simulink model "MAIN"  (R2021b)
settings: Solver=VariableStepAuto  StartTime=0.0  StopTime=10  RelTol=1e-3
undefined symbols (not defined in the file): c_Fuel, CM_FUEL_b, cmFuel_cmL, g, k_Fuel, L_TV, m_dot, m_iFuel, sigbuilder_block, T_min, VRfromNED_cordT, W_LANDER
libraries: matrix_library x3, slpidlib x2, shared6dof x1, simulink x1, aerolibanim x1, vrlib x1
settings Model: Creator=josepfamador  LastModifiedBy=josepfamador
settings DebuggingCC: SignalRangeChecking=warning  AlgebraicLoopMsg=none

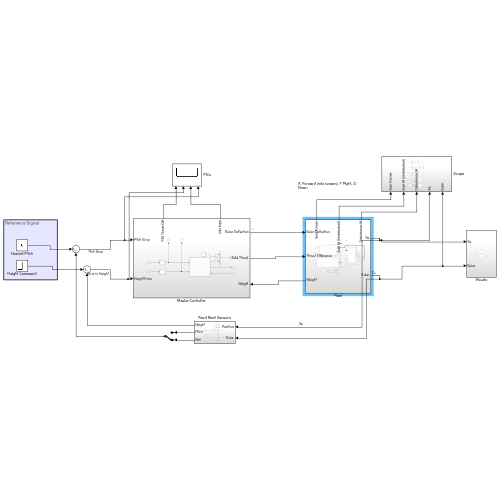
[thumbnail: Simulink's stored preview of the top-level diagram]
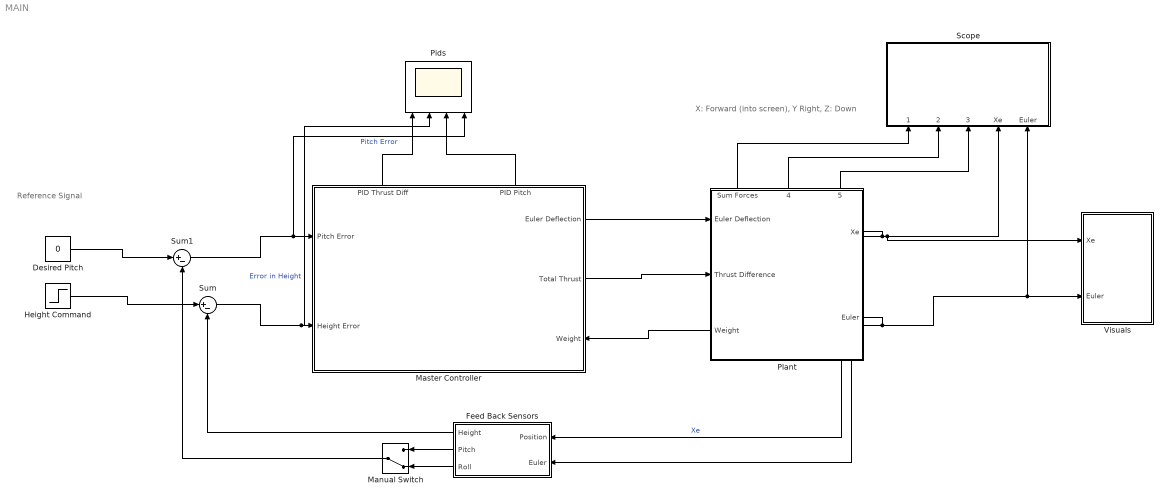
== system MAIN ==
  note: Reference Signal
  note: X: Forward (into screen), Y Right, Z: Down
  Desired Pitch : Constant  Value=0
  Feed Back Sensors : Subsystem
  Height Command : Step  SampleTime=0
  Manual Switch : ManualSwitch  CurrentSetting=0
  Master Controller : Subsystem
      settings: PortSchema="{\"entries\":[{\"content\":{\"sides\":[{\"content\":{\"connectorIds\":[\"In1\",\"In2\"]},\"type\":\"ConnectorPlacement.EquallySpacedRectSide\",\"uuid\":\"6b5f81e2-01db-4c59-bf08-4e3bf18bec3e\"},{\"content\":{\"connectorIds\":[\"Out1\",\"Out2\",\"In3\"],\"side\":\"RIGHT\"},\"type\":\"ConnectorPlacement.EquallySpacedRectSide\",\"uuid\":\"f97d49e1-5da4-4301-bd73-5a99c2855c55\"},{\"content\":{\"connectorIds\":[\"Out3\",\"Out4\"],\"side\":\"TOP\"},\"type\":\"ConnectorPlacement.EquallySpacedRectSide\",\"uuid\":\"d62bb92c-f39d-4cdf-a376-fbc7197c24fb\"}]},\"type\":\"ConnectorPlacement.EquallySpacedConnector\",\"uuid\":\"6638e0f7-5996-4093-84e0-c43993169f29\"}],\"packageUris\":[\"http://schema.mathworks.com/mf0/Connector/R2020b\"],\"version\":\"1.0\"}"
  Pids : Scope  NumInputPorts=4
  Plant : Subsystem
      settings: PortSchema="{\"entries\":[{\"content\":{\"sides\":[{\"content\":{\"connectorIds\":[\"In1\",\"In2\",\"Out6\"]},\"type\":\"ConnectorPlacement.EquallySpacedRectSide\",\"uuid\":\"a758654d-f9c5-4f69-af4d-6756fdff02ab\"},{\"content\":{\"connectorIds\":[\"Out1\",\"Out2\"],\"side\":\"RIGHT\"},\"type\":\"ConnectorPlacement.EquallySpacedRectSide\",\"uuid\":\"3ca0fdf4-fd7f-4f85-961a-cf19d643cdba\"},{\"content\":{\"connectorIds\":[\"Out3\",\"Out4\",\"Out5\"],\"side\":\"TOP\"},\"type\":\"ConnectorPlacement.EquallySpacedRectSide\",\"uuid\":\"8f9619ba-17bf-4a52-b197-69b799ce5fe6\"}]},\"type\":\"ConnectorPlacement.EquallySpacedConnector\",\"uuid\":\"48dcdf5d-501a-46a0-b089-89402a42e7cd\"}],\"packageUris\":[\"http://schema.mathworks.com/mf0/Connector/R2020b\"],\"version\":\"1.0\"}"
  Scope : Subsystem
  Sum : Sum  Inputs=|+-
  Sum1 : Sum  Inputs=|+-
  Visuals : Subsystem
  wires:
  Plant/1(Xe) -> Feed Back Sensors/1(Position), Scope/4(Xe), Visuals/1(Xe)  "Xe"
  Desired Pitch/1 -> Sum1/1
  Height Command/1 -> Sum/1
  Plant/2(Euler) -> Feed Back Sensors/2(Euler), Visuals/2(Euler), Scope/5(Euler)
  Feed Back Sensors/1(Height) -> Sum/2
  Sum1/1 -> Pids/4, Master Controller/1(Pitch Error)  "Pitch Error"
  Sum/1 -> Pids/2, Master Controller/2(Height Error)  "Error in Height"
  Plant/6(Weight) -> Master Controller/3(Weight)
  Master Controller/3(PID Thrust Diff) -> Pids/1
  Master Controller/4(PID Pitch) -> Pids/3
  Master Controller/1(Euler Deflection) -> Plant/1(Euler Deflection)
  Master Controller/2(Total Thrust) -> Plant/2(Thrust Difference)
  Plant/3(Sum Forces) -> Scope/1(Sum Forces)
  Plant/4(Sum M (Undisturbed)) -> Scope/2(Sum M (Undisturbed))
  Plant/5(Disturbance M) -> Scope/3(Disturbance M)
  Feed Back Sensors/3(Roll) -> Manual Switch/2
  Feed Back Sensors/2(Pitch) -> Manual Switch/1
  Manual Switch/1 -> Sum1/2

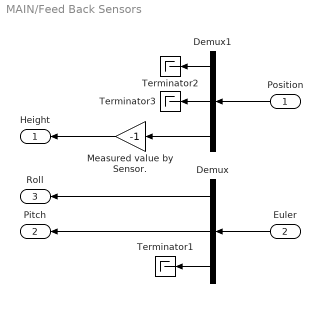
== system MAIN/Feed Back Sensors ==
  Position : Inport
  Euler : Inport  Port=2
  Demux : Demux  Outputs=3
  Demux1 : Demux  Outputs=3
  Measured value by Sensor. : Gain  Gain=-1
  Terminator1 : Terminator
  Terminator2 : Terminator
  Terminator3 : Terminator
  Height : Outport
  Pitch : Outport  Port=2
  Roll : Outport  Port=3
  wires:
  Position/1 -> Demux1/1
  Euler/1 -> Demux/1
  Measured value by Sensor./1 -> Height/1
  Demux/2 -> Pitch/1
  Demux/1 -> Roll/1
  Demux1/2 -> Terminator3/1
  Demux1/1 -> Terminator2/1
  Demux1/3 -> Measured value by Sensor./1
  Demux/3 -> Terminator1/1

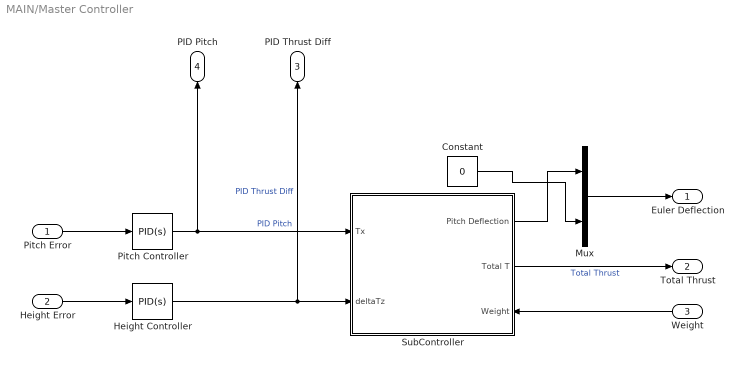
== system MAIN/Master Controller ==
  Pitch Error : Inport
  Height Error : Inport  Port=2
  Weight : Inport  Port=3
  Constant : Constant  Value=0
  Height Controller : slpidlib/PID Controller  Controller=PID  Form=Parallel  TimeDomain=Continuous-time  UseExternalTs=off  SampleTime=-1  IntegratorMethod=Forward Euler  FilterMethod=Forward Euler  ControllerParametersSource=internal  P=32  I=0.2  D=2  UseFilter=on  N=100  TunerSelectOption=Transfer Function Based (PID Tuner App)  InitialConditionSource=internal  InitialConditionForIntegrator=0  InitialConditionForFilter=0  DifferentiatorICPrevScaledInput=0  ExternalReset=none  TrackingMode=off  Kt=1  LimitOutput=on  SatLimitsSource=internal  UpperSaturationLimit=500  LowerSaturationLimit=-inf  LinearizeAsGain=off  AntiWindupMode=none  Kb=1  POutMin=[]  POutMax=[]  IOutMin=[]  IOutMax=[]  DOutMin=[]  DOutMax=[]  NOutMin=[]  NOutMax=[]  SumOutMin=[]  SumOutMax=[]  SaturationOutMin=[]  SaturationOutMax=[]  PParamMin=[]  PParamMax=[]  IParamMin=[]  IParamMax=[]  DParamMin=[]  DParamMax=[]  NParamMin=[]  NParamMax=[]  KbParamMin=[]  KbParamMax=[]  KtParamMin=[]  KtParamMax=[]  KbOutMin=[]  KbOutMax=[]  KtOutMin=[]  KtOutMax=[]  IntegratorOutMin=[]  IntegratorOutMax=[]  FilterOutMin=[]  FilterOutMax=[]  SumI1OutMin=[]  SumI1OutMax=[]  SumI2OutMin=[]  SumI2OutMax=[]  SumI3OutMin=[]  SumI3OutMax=[]  SumI4OutMin=[]  SumI4OutMax=[]  SumDOutMin=[]  SumDOutMax=[]  DifferentiatorOutMin=[]  DifferentiatorOutMax=[]  FilterDiffOutCoefMin=[]  FilterDiffOutCoefMax=[]  ReciprocalOutMin=[]  ReciprocalOutMax=[]  SumDenOutMin=[]  SumDenOutMax=[]  SumNumOutMin=[]  SumNumOutMax=[]  DivideOutMin=[]  DivideOutMax=[]  UdiffTsProdOutMin=[]  UdiffTsProdOutMax=[]  NTsProdOutMin=[]  NTsProdOutMax=[]  UintegralTsProdOutMin=[]  UintegralTsProdOutMax=[]  UngainTsProdOutMin=[]  UngainTsProdOutMax=[]  IntegratorContinuousStateAttributes=''  IntegratorStateMustResolveToSignalObject=off  IntegratorRTWStateStorageClass=Auto  FilterContinuousStateAttributes=''  FilterStateMustResolveToSignalObject=off  FilterRTWStateStorageClass=Auto  ParallelPVariant=InternalParameters  IdealPVariant=Disabled  IVariant=InternalParameters  DVariant=InternalParameters  IntegratorVariant=Continuous  SatVariant=Enabled  AWVariant=Passthrough  PCopyVariant=Disabled  TRVariant=Disabled  FdbkBlocksVariant=Forward  IdealPFdbkVariant=Disabled  SatFdbkVariant=Disabled  DerivativeFilterVariant=ContFilter  NVariant=InternalParameters  NCopyVariant=Disabled  FilterICVariant=InternalICsFilter  IntegratorICVariant=InternalICs  ExternalResetVariant=Disabled  TRSumVariant=Passthrough  SumFdbkVariant=Disabled  SumVariant=Sum_PID  TsampFilterVariant=InternalTs  TsampNgainVariant=Passthrough  TsampIntegralVariant=Passthrough  ExternalSaturationOutDataTypeStr=Inherit: Same as second input
  Mux : Mux  Inputs=2
  Pitch Controller : slpidlib/PID Controller  Controller=PID  Form=Parallel  TimeDomain=Continuous-time  UseExternalTs=off  SampleTime=-1  IntegratorMethod=Forward Euler  FilterMethod=Forward Euler  ControllerParametersSource=internal  P=-0.5002  I=0  D=0  UseFilter=on  N=100  TunerSelectOption=Frequency Response Based  InitialConditionSource=internal  InitialConditionForIntegrator=0  InitialConditionForFilter=0  DifferentiatorICPrevScaledInput=0  ExternalReset=none  TrackingMode=off  Kt=1  LimitOutput=on  SatLimitsSource=internal  UpperSaturationLimit=0.2618  LowerSaturationLimit=-0.2618  LinearizeAsGain=on  AntiWindupMode=none  Kb=1  POutMin=[]  POutMax=[]  IOutMin=[]  IOutMax=[]  DOutMin=[]  DOutMax=[]  NOutMin=[]  NOutMax=[]  SumOutMin=[]  SumOutMax=[]  SaturationOutMin=[]  SaturationOutMax=[]  PParamMin=[]  PParamMax=[]  IParamMin=[]  IParamMax=[]  DParamMin=[]  DParamMax=[]  NParamMin=[]  NParamMax=[]  KbParamMin=[]  KbParamMax=[]  KtParamMin=[]  KtParamMax=[]  KbOutMin=[]  KbOutMax=[]  KtOutMin=[]  KtOutMax=[]  IntegratorOutMin=[]  IntegratorOutMax=[]  FilterOutMin=[]  FilterOutMax=[]  SumI1OutMin=[]  SumI1OutMax=[]  SumI2OutMin=[]  SumI2OutMax=[]  SumI3OutMin=[]  SumI3OutMax=[]  SumI4OutMin=[]  SumI4OutMax=[]  SumDOutMin=[]  SumDOutMax=[]  DifferentiatorOutMin=[]  DifferentiatorOutMax=[]  FilterDiffOutCoefMin=[]  FilterDiffOutCoefMax=[]  ReciprocalOutMin=[]  ReciprocalOutMax=[]  SumDenOutMin=[]  SumDenOutMax=[]  SumNumOutMin=[]  SumNumOutMax=[]  DivideOutMin=[]  DivideOutMax=[]  UdiffTsProdOutMin=[]  UdiffTsProdOutMax=[]  NTsProdOutMin=[]  NTsProdOutMax=[]  UintegralTsProdOutMin=[]  UintegralTsProdOutMax=[]  UngainTsProdOutMin=[]  UngainTsProdOutMax=[]  IntegratorContinuousStateAttributes=''  IntegratorStateMustResolveToSignalObject=off  IntegratorRTWStateStorageClass=Auto  FilterContinuousStateAttributes=''  FilterStateMustResolveToSignalObject=off  FilterRTWStateStorageClass=Auto  ParallelPVariant=InternalParameters  IdealPVariant=Disabled  IVariant=InternalParameters  DVariant=InternalParameters  IntegratorVariant=Continuous  SatVariant=Enabled  AWVariant=Passthrough  PCopyVariant=Disabled  TRVariant=Disabled  FdbkBlocksVariant=Forward  IdealPFdbkVariant=Disabled  SatFdbkVariant=Disabled  DerivativeFilterVariant=ContFilter  NVariant=InternalParameters  NCopyVariant=Disabled  FilterICVariant=InternalICsFilter  IntegratorICVariant=InternalICs  ExternalResetVariant=Disabled  TRSumVariant=Passthrough  SumFdbkVariant=Disabled  SumVariant=Sum_PID  TsampFilterVariant=InternalTs  TsampNgainVariant=Passthrough  TsampIntegralVariant=Passthrough  ExternalSaturationOutDataTypeStr=Inherit: Same as second input
  SubController : Subsystem
      settings: PortSchema="{\"entries\":[{\"content\":{\"sides\":[{\"content\":{\"connectorIds\":[\"In1\",\"In2\"]},\"type\":\"ConnectorPlacement.EquallySpacedRectSide\",\"uuid\":\"09ce5825-295e-43a7-9644-a5328231df2c\"},{\"content\":{\"connectorIds\":[\"Out1\",\"Out2\",\"In3\"],\"side\":\"RIGHT\"},\"type\":\"ConnectorPlacement.EquallySpacedRectSide\",\"uuid\":\"578e798d-aacd-4cff-b78a-042079318f31\"},{\"content\":{\"connectorIds\":[],\"side\":\"TOP\"},\"type\":\"ConnectorPlacement.EquallySpacedRectSide\",\"uuid\":\"66791839-dddf-41e6-aa5f-32841b466e1e\"}]},\"type\":\"ConnectorPlacement.EquallySpacedConnector\",\"uuid\":\"3e01a88c-8ac0-4240-97e5-f19006a6fa45\"}],\"packageUris\":[\"http://schema.mathworks.com/mf0/Connector/R2020b\"],\"version\":\"1.0\"}"
  Euler Deflection : Outport
  Total Thrust : Outport  Port=2
  PID Thrust Diff : Outport  Port=3
  PID Pitch : Outport  Port=4
  wires:
  Mux/1 -> Euler Deflection/1
  Height Error/1 -> Height Controller/1
  Weight/1 -> SubController/3(Weight)
  SubController/2(Total T) -> Total Thrust/1  "Total Thrust"
  Height Controller/1 -> SubController/2(deltaTz), PID Thrust Diff/1  "PID Thrust Diff"
  Pitch Controller/1 -> SubController/1(Tx), PID Pitch/1  "PID Pitch"
  Pitch Error/1 -> Pitch Controller/1
  SubController/1(Pitch Deflection) -> Mux/1
  Constant/1 -> Mux/2

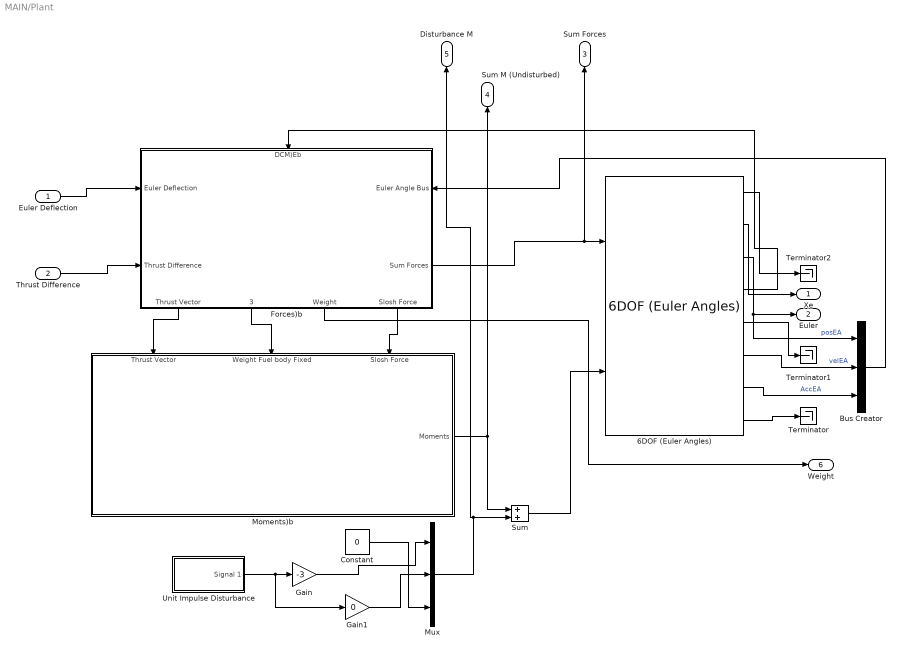
== system MAIN/Plant ==
  Euler Deflection : Inport
  Thrust Difference : Inport  Port=2
  6DOF (Euler Angles) : shared6dof/6DOF (Euler Angles)  units=Metric (MKS)  mtype=Fixed  rep=Euler Angles  xme_0=[0 0 0]  Vm_0=[0 0 0]  eul_0=[0 0 0]  pm_0=[0 0 0]  mass_0=M_lander  mass_e=0.5  mass_f=2.0  inertia=I  inertia_e=eye(3)  inertia_f=2*eye(3)  k_quat=1.0  vre_flag=on  abi_flag=off  aMode=0  xme_statename=''  Vm_statename=''  eul_statename=''  quat_statename=''  pm_statename=''  mass_statename=''
      settings: SourceProductBaseCode=AE,PW,DR,MT,UV,VE
  Bus Creator : BusCreator  Inputs=3
  Constant : Constant  Value=0
  Forces)b : Subsystem
      settings: PortSchema="{\"entries\":[{\"content\":{\"sides\":[{\"content\":{\"connectorIds\":[\"In1\",\"In2\"]},\"type\":\"ConnectorPlacement.EquallySpacedRectSide\",\"uuid\":\"f2cd2bb8-6e5d-4153-a512-e15a3f9d81c4\"},{\"content\":{\"connectorIds\":[\"In4\",\"Out1\"],\"side\":\"RIGHT\"},\"type\":\"ConnectorPlacement.EquallySpacedRectSide\",\"uuid\":\"118a6529-12fa-490e-97a8-013bcc90e0c4\"},{\"content\":{\"connectorIds\":[\"In3\"],\"side\":\"TOP\"},\"type\":\"ConnectorPlacement.EquallySpacedRectSide\",\"uuid\":\"99a35966-8420-41f8-be1a-036ce80ff0d6\"},{\"content\":{\"connectorIds\":[\"Out2\",\"Out3\",\"Out4\",\"Out5\"],\"side\":\"BOTTOM\"},\"type\":\"ConnectorPlacement.EquallySpacedRectSide\",\"uuid\":\"85926175-8560-4c6d-bfea-5508daccda47\"}]},\"type\":\"ConnectorPlacement.EquallySpacedConnector\",\"uuid\":\"17491b4d-b23c-405f-97c9-eb7c998e3d68\"}],\"packageUris\":[\"http://schema.mathworks.com/mf0/Connector/R2020b\"],\"version\":\"1.0\"}"
  Gain : Gain  Gain=-3
  Gain1 : Gain  Gain=0
  Moments)b : Subsystem
      settings: PortSchema="{\"entries\":[{\"content\":{\"sides\":[{\"content\":{\"connectorIds\":[]},\"type\":\"ConnectorPlacement.EquallySpacedRectSide\",\"uuid\":\"57bc3e64-de08-407a-928b-1dcbce02ca7d\"},{\"content\":{\"connectorIds\":[\"Out1\"],\"side\":\"RIGHT\"},\"type\":\"ConnectorPlacement.EquallySpacedRectSide\",\"uuid\":\"aa88f6e7-8b22-4f67-9b59-e952a02f1ee1\"},{\"content\":{\"connectorIds\":[\"In1\",\"In2\",\"In3\"],\"side\":\"TOP\"},\"type\":\"ConnectorPlacement.EquallySpacedRectSide\",\"uuid\":\"5b52c472-2b0f-4159-8979-6365ad52eb05\"}]},\"type\":\"ConnectorPlacement.EquallySpacedConnector\",\"uuid\":\"cac2b4e7-f15a-4ffc-9b20-68f1334fb4cb\"}],\"packageUris\":[\"http://schema.mathworks.com/mf0/Connector/R2020b\"],\"version\":\"1.0\"}"
  Mux : Mux  Inputs=3
  Sum : Sum
  Terminator : Terminator
  Terminator1 : Terminator
  Terminator2 : Terminator
  Unit Impulse Disturbance : Subsystem  Tag=STV Subsys  LoadFcn=sigbuilder_block('load');  StartFcn=sigbuilder_block('start');  StopFcn=sigbuilder_block('stop');  ClipboardFcn=sigbuilder_block('clipboard');  mask(Sigbuilder block){tuvar=[0:10]}
      mask help: Simulink:masks:SigbuilderBlock_MD
      mask init:
      | if ~strcmp(get_param(bdroot(gcbh),'SimulationStatus'),'stopped') tuvar = sigbuilder_block('maskInit'); end
      settings: CopyFcn=sigbuilder_block('copy');  DeleteFcn=sigbuilder_block('delete');  ModelCloseFcn=sigbuilder_block('modelClose');  PreSaveFcn=sigbuilder_block('preSave');  PauseFcn=sigbuilder_block('pause');  ContinueFcn=sigbuilder_block('continue');  NameChangeFcn=sigbuilder_block('namechange');  OpenFcn=sigbuilder_block('open',[204 256 550 400 ]);  CloseFcn=sigbuilder_block('close');
      mask Display: plot(0, 0, 100, 100,[2, 2, 32, 32, 2], [68, 8, 8, 68, 68],[32, 2], [38, 38], [32, 19, 2],[53, 60, 44], [32, 17, 17, 2],[16, 16, 31, 31]);txt = getActiveGroup(gcbh);text(2, 100, txt,'verticalAlignment', 'top');
  Xe : Outport
  Euler : Outport  Port=2
  Sum Forces : Outport  Port=3
  Sum M (Undisturbed) : Outport  Port=4
  Disturbance M : Outport  Port=5
  Weight : Outport  Port=6
  wires:
  6DOF (Euler Angles)/6 -> Bus Creator/2  "velEA"
  6DOF (Euler Angles)/3 -> Euler/1, Bus Creator/1  "posEA"
  6DOF (Euler Angles)/2 -> Xe/1
  6DOF (Euler Angles)/7 -> Bus Creator/3  "AccEA"
  Euler Deflection/1 -> Forces)b/1(Euler Deflection)
  Thrust Difference/1 -> Forces)b/2(Thrust Difference)
  6DOF (Euler Angles)/4 -> Forces)b/3(DCM)Eb)
  Bus Creator/1 -> Forces)b/4(Euler Angle Bus)
  Forces)b/3(WeightFuel)bodyFixed) -> Moments)b/2(Weight Fuel body Fixed)
  Forces)b/2(Thrust Vector) -> Moments)b/1(Thrust Vector)
  6DOF (Euler Angles)/8 -> Terminator/1
  6DOF (Euler Angles)/5 -> Terminator1/1
  6DOF (Euler Angles)/1 -> Terminator2/1
  Forces)b/4(Weight) -> Weight/1
  Moments)b/1(Moments) -> Sum/1, Sum M (Undisturbed)/1
  Sum/1 -> 6DOF (Euler Angles)/2
  Forces)b/5(Slosh Force) -> Moments)b/3(Slosh Force)
  Forces)b/1(Sum Forces) -> Sum Forces/1, 6DOF (Euler Angles)/1
  Mux/1 -> Disturbance M/1, Sum/2
  Unit Impulse Disturbance/1(Signal 1) -> Gain1/1, Gain/1
  Gain/1 -> Mux/1
  Gain1/1 -> Mux/2
  Constant/1 -> Mux/3

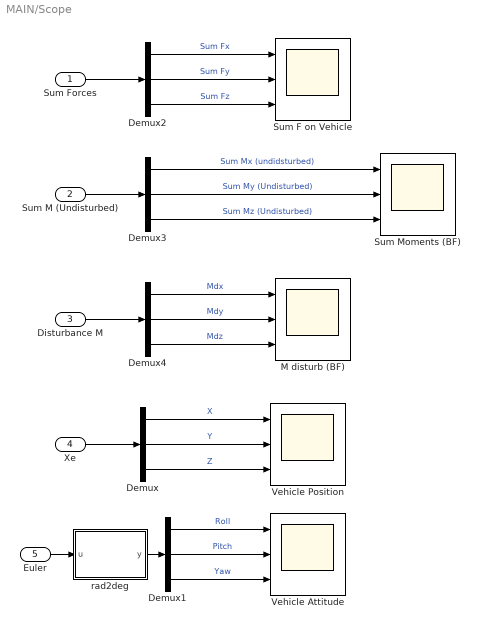
== system MAIN/Scope ==
  Sum Forces : Inport
  Sum M (Undisturbed) : Inport  Port=2
  Disturbance M : Inport  Port=3
  Xe : Inport  Port=4
  Euler : Inport  Port=5
  Demux{,1..4} (5 alike) : Demux  Outputs=3
  M disturb (BF) : Scope  NumInputPorts=3
  Sum F on Vehicle : Scope  NumInputPorts=3
  Sum Moments (BF) : Scope  NumInputPorts=3
  Vehicle Attitude : Scope  NumInputPorts=3
  Vehicle Position : Scope  NumInputPorts=3
  rad2deg : MATLAB Function  TreatAsAtomicUnit=on
  wires:
  Xe/1 -> Demux/1
  Demux/2 -> Vehicle Position/2  "Y"
  Demux/1 -> Vehicle Position/1  "X"
  Demux/3 -> Vehicle Position/3  "Z"
  Euler/1 -> rad2deg/1(u)
  Demux1/1 -> Vehicle Attitude/1  "Roll"
  Demux1/2 -> Vehicle Attitude/2  "Pitch"
  Demux1/3 -> Vehicle Attitude/3  "Yaw"
  Demux2/2 -> Sum F on Vehicle/2  "Sum Fy"
  Demux2/1 -> Sum F on Vehicle/1  "Sum Fx"
  Sum Forces/1 -> Demux2/1
  Demux2/3 -> Sum F on Vehicle/3  "Sum Fz"
  Demux3/1 -> Sum Moments (BF)/1  "Sum Mx (undidsturbed)"
  Sum M (Undisturbed)/1 -> Demux3/1
  Demux3/3 -> Sum Moments (BF)/3  "Sum Mz (Undisturbed)"
  Demux3/2 -> Sum Moments (BF)/2  "Sum My (Undisturbed)"
  Demux4/1 -> M disturb (BF)/1  "Mdx"
  Disturbance M/1 -> Demux4/1
  Demux4/3 -> M disturb (BF)/3  "Mdz"
  Demux4/2 -> M disturb (BF)/2  "Mdy"
  rad2deg/1(y) -> Demux1/1

== system MAIN/Visuals ==
  Xe : Inport
  Euler : Inport  Port=2
  6DoF Animation1 : aerolibanim/6DoF Animation  u1=[-5 5 -5 5 0 4]  u2=0.1  u3=1  u4=[0 0 -1]  u5=Fixed position  u6=[-10 0 0]  u7=45  u8=off
  Coord Transforms : Subsystem
  VR Sink : vrlib/VR Sink  InstantiateOnLoad=on  SampleTime=-1  ViewEnable=on  RemoteChange=off  RemoteView=off  FieldsWritten=Lander.rotation.4.1.1.double#Lander.translation.3.1.1.double  WorldFileName=/Users/josepfamador/RPL_controls/vrsinkstuff/V6b.x3d  AutoView=off  VideoDimensions=[]  AllowVariableSize=off  FigureProperties="{'Position', 'Name', 'Viewpoint', 'CameraBound', 'CameraDirection', 'CameraPosition', 'CameraUpVector', 'ZoomFactor', 'Antialiasing', 'Headlight', 'Lighting', 'NavPanel', 'Sound', 'StatusBar', 'Stereo3D', 'Stereo3DCameraOffset', 'Stereo3DHIT', 'ToolBar', 'Textures', 'Transparency', 'Triad', 'Wireframe', 'NavZones', 'NavMode', 'NavSpeed', 'CaptureFileFormat', 'CaptureFileName', 'Record2DCompressMethod', 'Record2DCompressQuality', 'Record2D', 'Record2DFileName', 'Record2DFPS'; [4.3300000000000000e+02   4.8400000000000000e+02   1.0600000000000000e+03   6.6800000000000000e+02], '', '_untitled_1', 'on', [0.0000000000000000e+00   0.0000000000000000e+00  -1.0000000000000000e+00], [0.0000000000000000e+00   0.0000000000000000e+00   0.0000000000000000e+00], [0.0000000000000000e+00   1.0000000000000000e+00   0.0000000000000000e+00], [1.0000000000000000e+00], 'on', 'on', 'on', 'minimized', 'on', 'on', 'off', [1.0000000149011612e-01], [0.0000000000000000e+00], 'on', 'on', 'on', 'none', 'off', 'off', 'fly', 'normal', 'tif', '%f_anim_%n.tif', 'auto', [7.5000000000000000e+01], 'off', '%f_anim_%n.avi', 'auto'}"
  wires:
  Euler/1 -> 6DoF Animation1/2, Coord Transforms/1(eulers)
  Coord Transforms/2(VR Translation) -> VR Sink/2
  Coord Transforms/1(VR Rotation) -> VR Sink/1
  Xe/1 -> 6DoF Animation1/1, Coord Transforms/2(Earth Body Position)

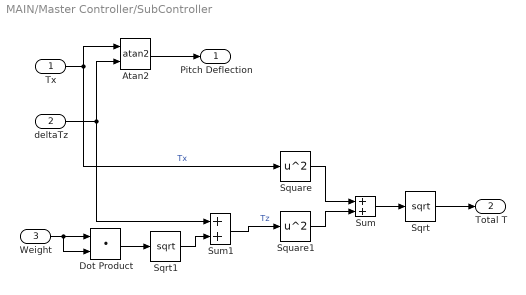
== system MAIN/Master Controller/SubController ==
  Tx : Inport
  deltaTz : Inport  Port=2
  Weight : Inport  Port=3
  Atan2 : Trigonometry  Operator=atan2
  Dot Product : DotProduct  InputSameDT=on  OutDataTypeStr=Inherit: Inherit via internal rule
  Sqrt : Sqrt  SaturateOnIntegerOverflow=on
  Sqrt1 : Sqrt  SaturateOnIntegerOverflow=on
  Square : Math  Operator=square  SaturateOnIntegerOverflow=on
  Square1 : Math  Operator=square  SaturateOnIntegerOverflow=on
  Sum : Sum
  Sum1 : Sum
  Pitch Deflection : Outport
  Total T : Outport  Port=2
  wires:
  Tx/1 -> Square/1, Atan2/1  "Tx"
  deltaTz/1 -> Sum1/1, Atan2/2
  Atan2/1 -> Pitch Deflection/1
  Square/1 -> Sum/1
  Sum1/1 -> Square1/1  "Tz"
  Sum/1 -> Sqrt/1
  Sqrt/1 -> Total T/1
  Weight/1 -> Dot Product/2, Dot Product/1
  Sqrt1/1 -> Sum1/2
  Dot Product/1 -> Sqrt1/1
  Square1/1 -> Sum/2

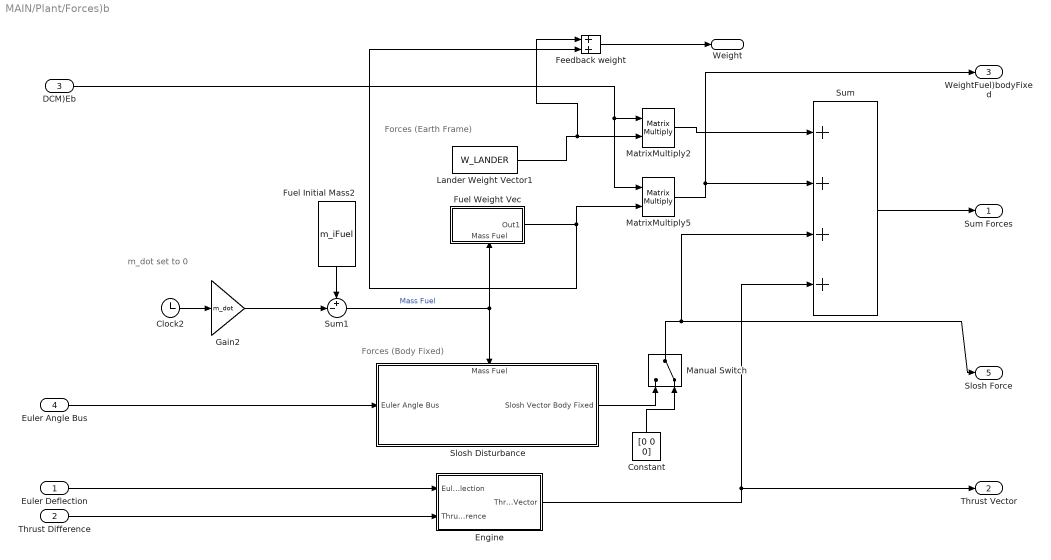
== system MAIN/Plant/Forces)b ==
  note: m_dot set to 0
  note: Forces (Earth Frame)
  note: Forces (Body Fixed)
  Euler Deflection : Inport
  Thrust Difference : Inport  Port=2
  DCM)Eb : Inport  Port=3
  Euler Angle Bus : Inport  Port=4
  Clock2 : Clock
  Constant : Constant  Value=[0 0 0]
  Engine : Subsystem
  Feedback weight : Sum
  Fuel Initial Mass2 : Constant  Value=m_iFuel
  Fuel Weight Vec : Subsystem
      settings: PortSchema="{\"entries\":[{\"content\":{\"sides\":[{\"content\":{\"connectorIds\":[]},\"type\":\"ConnectorPlacement.EquallySpacedRectSide\",\"uuid\":\"3ac8771b-a081-406d-94b3-c49ccf45ccde\"},{\"content\":{\"connectorIds\":[\"Out1\"],\"side\":\"RIGHT\"},\"type\":\"ConnectorPlacement.EquallySpacedRectSide\",\"uuid\":\"be409403-c355-43ab-922f-674d94fb1088\"},{\"content\":{\"connectorIds\":[],\"side\":\"TOP\"},\"type\":\"ConnectorPlacement.EquallySpacedRectSide\",\"uuid\":\"5154e291-8627-43d1-b53a-1bb36ae892a9\"},{\"content\":{\"connectorIds\":[\"In1\"],\"side\":\"BOTTOM\"},\"type\":\"ConnectorPlacement.EquallySpacedRectSide\",\"uuid\":\"de6d836d-8ff3-44c1-9409-8d936df793a7\"}]},\"type\":\"ConnectorPlacement.EquallySpacedConnector\",\"uuid\":\"c160a2b3-10aa-447d-ad60-2ea5b4c61963\"}],\"packageUris\":[\"http://schema.mathworks.com/mf0/Connector/R2020b\"],\"version\":\"1.0\"}"
  Gain2 : Gain  Gain=m_dot
  Lander Weight Vector1 : Constant  Value=W_LANDER
  Manual Switch : ManualSwitch  CurrentSetting=0
  MatrixMultiply2 : Product  Multiplication=Matrix(*)
  MatrixMultiply5 : Product  Multiplication=Matrix(*)
  Slosh Disturbance : Subsystem
      settings: PortSchema="{\"entries\":[{\"content\":{\"sides\":[{\"content\":{\"connectorIds\":[\"In1\"]},\"type\":\"ConnectorPlacement.EquallySpacedRectSide\",\"uuid\":\"57bc3e64-de08-407a-928b-1dcbce02ca7d\"},{\"content\":{\"connectorIds\":[\"Out1\"],\"side\":\"RIGHT\"},\"type\":\"ConnectorPlacement.EquallySpacedRectSide\",\"uuid\":\"aa88f6e7-8b22-4f67-9b59-e952a02f1ee1\"},{\"content\":{\"connectorIds\":[\"In2\"],\"side\":\"TOP\"},\"type\":\"ConnectorPlacement.EquallySpacedRectSide\",\"uuid\":\"5b52c472-2b0f-4159-8979-6365ad52eb05\"}]},\"type\":\"ConnectorPlacement.EquallySpacedConnector\",\"uuid\":\"cac2b4e7-f15a-4ffc-9b20-68f1334fb4cb\"}],\"packageUris\":[\"http://schema.mathworks.com/mf0/Connector/R2020b\"],\"version\":\"1.0\"}"
  Sum : Sum  Inputs=++++
  Sum1 : Sum  Inputs=+-|
  Sum Forces : Outport
  Thrust Vector : Outport  Port=2
  WeightFuel)bodyFixed : Outport  Port=3
  Weight : Outport  Port=4
  Slosh Force : Outport  Port=5
  wires:
  Sum/1 -> Sum Forces/1
  Euler Angle Bus/1 -> Slosh Disturbance/1(Euler Angle Bus)
  Gain2/1 -> Sum1/2
  Clock2/1 -> Gain2/1
  Sum1/1 -> Fuel Weight Vec/1(Mass Fuel), Slosh Disturbance/2(Mass Fuel)  "Mass Fuel"
  MatrixMultiply2/1 -> Sum/1
  Engine/1(Thrust Vector) -> Sum/4, Thrust Vector/1
  Fuel Weight Vec/1(Out1) -> MatrixMultiply5/2, Feedback weight/2
  Slosh Disturbance/1(Slosh Vector Body Fixed) -> Manual Switch/1
  Euler Deflection/1 -> Engine/1(Euler Deflection)
  Thrust Difference/1 -> Engine/2(Thrust Difference)
  Fuel Initial Mass2/1 -> Sum1/1
  Lander Weight Vector1/1 -> Feedback weight/1, MatrixMultiply2/2
  MatrixMultiply5/1 -> WeightFuel)bodyFixed/1, Sum/2
  DCM)Eb/1 -> MatrixMultiply5/1, MatrixMultiply2/1
  Feedback weight/1 -> Weight/1
  Constant/1 -> Manual Switch/2
  Manual Switch/1 -> Sum/3, Slosh Force/1

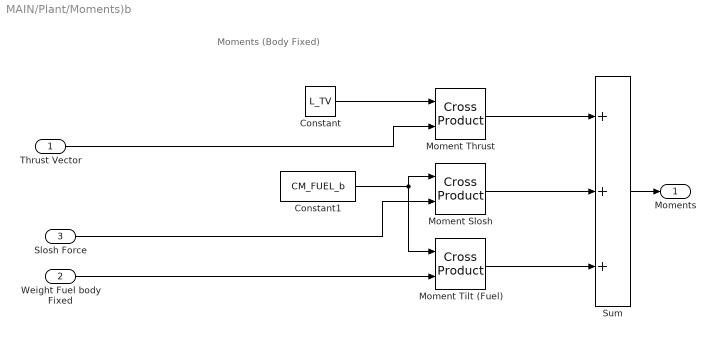
== system MAIN/Plant/Moments)b ==
  note: Moments (Body Fixed)
  Thrust Vector : Inport
  Weight Fuel body Fixed : Inport  Port=2
  Slosh Force : Inport  Port=3
  Constant : Constant  Value=L_TV
  Constant1 : Constant  Value=CM_FUEL_b
  Moment Slosh : matrix_library/Cross Product
      settings: SourceProductBaseCode=SL
  Moment Thrust : matrix_library/Cross Product
      settings: SourceProductBaseCode=SL
  Moment Tilt (Fuel) : matrix_library/Cross Product
      settings: SourceProductBaseCode=SL
  Sum : Sum  Inputs=+++
  Moments : Outport
  wires:
  Sum/1 -> Moments/1
  Thrust Vector/1 -> Moment Thrust/2
  Constant/1 -> Moment Thrust/1
  Constant1/1 -> Moment Tilt (Fuel)/1, Moment Slosh/1
  Moment Thrust/1 -> Sum/1
  Moment Slosh/1 -> Sum/2
  Weight Fuel body Fixed/1 -> Moment Tilt (Fuel)/2
  Moment Tilt (Fuel)/1 -> Sum/3
  Slosh Force/1 -> Moment Slosh/2

== system MAIN/Plant/Unit Impulse Disturbance ==
  Demux : Demux  Tag=STV Demux  Outputs=1
      settings: DisplayOption=none
  FromWs : FromWorkspace  Tag=STV FromWs  VariableName=tuvar
      SigBuilderData=|
      | common.afterFinalStr = 'Extrapolate'
      | common.sampleTime = 0
      | dataSet.timeRange = [0 10]
      | dataSet.name = 'Group 1'
      | sbobj.Groups.Name = 'Group 1'
      | sbobj.Groups.Signals.Name = 'Signal 1'
      | sbobj.Groups.Signals.XData = [0 1.45 1.45 1.4895 1.4895 10]
      | sbobj.Groups.Signals.YData = [0 0 1 1 0 0]
  Signal 1 : Outport  Tag=STV Outport
  wires:
  Demux/1 -> Signal 1/1
  FromWs/1 -> Demux/1

== system MAIN/Visuals/Coord Transforms ==
  eulers : Inport
  Earth Body Position : Inport  Port=2
  Constant1 : Constant  Value=VRfromNED_cordT
  Generalized Principle Axis and Angle of Rotation : MATLAB Function  TreatAsAtomicUnit=on
  MatrixMultiply : Product  Multiplication=Matrix(*)
  Mux1 : Mux  Inputs=2
  NED Euler to VR Euler : MATLAB Function  TreatAsAtomicUnit=on
  VR Rotation : Outport
  VR Translation : Outport  Port=2
  wires:
  Mux1/1 -> VR Rotation/1  "VR Axis and Rot"
  Earth Body Position/1 -> MatrixMultiply/2
  MatrixMultiply/1 -> VR Translation/1
  NED Euler to VR Euler/1(C) -> Generalized Principle Axis and Angle of Rotation/1(RotMat)
  eulers/1 -> NED Euler to VR Euler/1(eu)
  Generalized Principle Axis and Angle of Rotation/1(A) -> Mux1/1
  Generalized Principle Axis and Angle of Rotation/2(phi) -> Mux1/2
  Constant1/1 -> MatrixMultiply/1

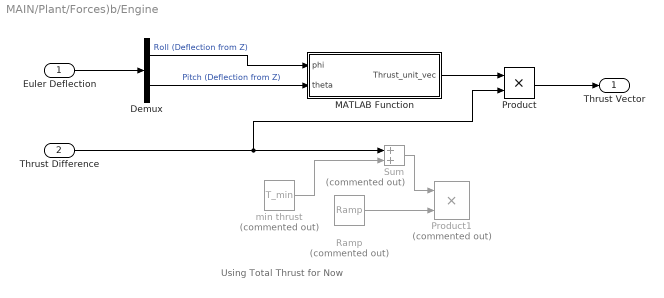
== system MAIN/Plant/Forces)b/Engine ==
  note: Using Total Thrust for Now
  Euler Deflection : Inport
  Thrust Difference : Inport  Port=2
  Demux : Demux  Outputs=2
  MATLAB Function : MATLAB Function  TreatAsAtomicUnit=on
  Product : Product
  Product1 : Product  Commented=on
  Ramp : simulink/Sources/Ramp  Commented=on  slope=0.01  start=0.5  InitialOutput=1
  Sum : Sum  Commented=on
  min thrust : Constant  Commented=on  Value=T_min
  Thrust Vector : Outport
  wires:
  Euler Deflection/1 -> Demux/1
  Thrust Difference/1 -> Product/2, Sum/1
  min thrust/1 -> Sum/2
  Demux/1 -> MATLAB Function/1(phi)  "Roll (Deflection from Z)"
  Demux/2 -> MATLAB Function/2(theta)  "Pitch (Deflection from Z)"
  MATLAB Function/1(Thrust_unit_vec) -> Product/1
  Sum/1 -> Product1/1
  Product/1 -> Thrust Vector/1
  Ramp/1 -> Product1/2

== system MAIN/Plant/Forces)b/Fuel Weight Vec ==
  Mass Fuel : Inport
  Constant1 : Constant  Value=0
  Constant8 : Constant  Value=0
  Gain1 : Gain  Gain=g
  Some Mux : Mux  Inputs=3
  Out1 : Outport
  wires:
  Constant8/1 -> Some Mux/1
  Gain1/1 -> Some Mux/3  "Weight_Fuel"
  Constant1/1 -> Some Mux/2
  Some Mux/1 -> Out1/1
  Mass Fuel/1 -> Gain1/1

== system MAIN/Plant/Forces)b/Slosh Disturbance ==
  Euler Angle Bus : Inport
  Mass Fuel : Inport  Port=2
  0 disturbance in Z body fixed frmae : Constant  Value=0
  Constant : Constant  Value=cmFuel_cmL
  Euler Angle Splitter : Subsystem
  Mass Force in x_b : Subsystem
  Mass Force in y_b : Subsystem
  Mux : Mux  Inputs=3
  Slosh Vector Body Fixed : Outport
  wires:
  Constant/1 -> Mass Force in y_b/3(Arm_length r), Mass Force in x_b/3(Arm_length r)
  Mass Fuel/1 -> Mass Force in y_b/1(Mass), Mass Force in x_b/1(Mass)
  Euler Angle Bus/1 -> Euler Angle Splitter/1(Euler Angle Bus)
  Mass Force in x_b/1(Disturbance_x_b) -> Mux/1
  Euler Angle Splitter/1("phi, phi_d, phi_2d") -> Mass Force in y_b/2("Ang, d, 2d")
  Mass Force in y_b/1(Disturbance_y_b) -> Mux/2
  Euler Angle Splitter/2(theta,theta_d,theta_2d) -> Mass Force in x_b/2("Ang, d, 2d")
  0 disturbance in Z body fixed frmae/1 -> Mux/3
  Mux/1 -> Slosh Vector Body Fixed/1

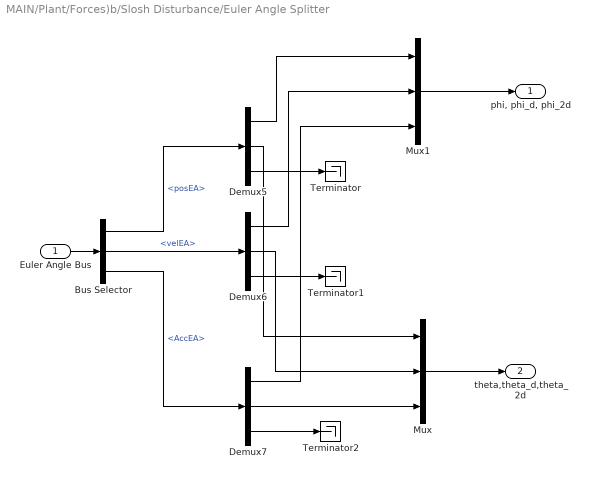
== system MAIN/Plant/Forces)b/Slosh Disturbance/Euler Angle Splitter ==
  Euler Angle Bus : Inport
  Bus Selector : BusSelector  OutputSignals=posEA,velEA,AccEA
  Demux5 : Demux  Outputs=3
  Demux6 : Demux  Outputs=3
  Demux7 : Demux  Outputs=3
  Mux : Mux  Inputs=3
  Mux1 : Mux  Inputs=3
  Terminator : Terminator
  Terminator1 : Terminator
  Terminator2 : Terminator
  "phi, phi_d, phi_2d" : Outport
  theta,theta_d,theta_2d : Outport  Port=2
  wires:
  Demux5/2 -> Mux/1
  Demux6/2 -> Mux/2
  Demux7/2 -> Mux/3
  Mux/1 -> theta,theta_d,theta_2d/1
  Demux5/1 -> Mux1/1
  Demux6/1 -> Mux1/2
  Demux7/1 -> Mux1/3
  Mux1/1 -> "phi, phi_d, phi_2d"/1
  Demux5/3 -> Terminator/1
  Demux6/3 -> Terminator1/1
  Demux7/3 -> Terminator2/1
  Euler Angle Bus/1 -> Bus Selector/1
  Bus Selector/1 -> Demux5/1  "<posEA>"
  Bus Selector/2 -> Demux6/1  "<velEA>"
  Bus Selector/3 -> Demux7/1  "<AccEA>"

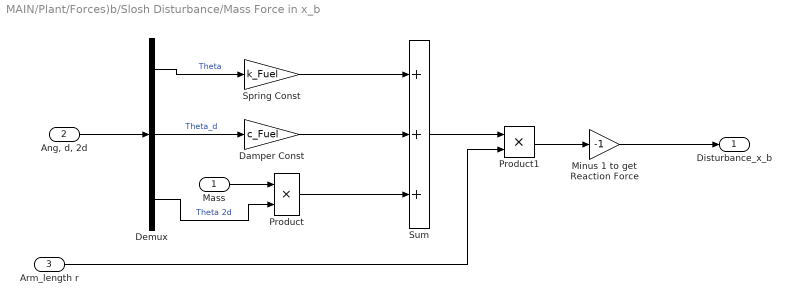
== system MAIN/Plant/Forces)b/Slosh Disturbance/Mass Force in x_b ==
  Mass : Inport
  "Ang, d, 2d" : Inport  Port=2
  Arm_length r : Inport  Port=3
  Damper Const : Gain  Gain=c_Fuel
  Demux : Demux  Outputs=3
  Minus 1 to get Reaction Force : Gain  Gain=-1
  Product : Product
  Product1 : Product
  Spring Const : Gain  Gain=k_Fuel
  Sum : Sum  Inputs=+++
  Disturbance_x_b : Outport
  wires:
  Mass/1 -> Product/1
  Spring Const/1 -> Sum/1
  Damper Const/1 -> Sum/2
  Product/1 -> Sum/3
  Sum/1 -> Product1/1
  Arm_length r/1 -> Product1/2
  Product1/1 -> Minus 1 to get Reaction Force/1
  Minus 1 to get Reaction Force/1 -> Disturbance_x_b/1
  "Ang, d, 2d"/1 -> Demux/1
  Demux/1 -> Spring Const/1  "Theta"
  Demux/2 -> Damper Const/1  "Theta_d"
  Demux/3 -> Product/2  "Theta 2d"

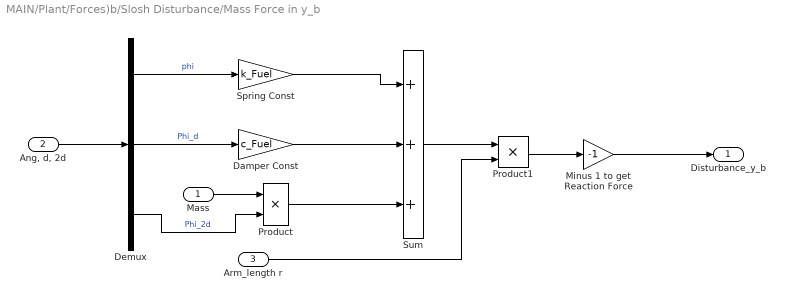
== system MAIN/Plant/Forces)b/Slosh Disturbance/Mass Force in y_b ==
  Mass : Inport
  "Ang, d, 2d" : Inport  Port=2
  Arm_length r : Inport  Port=3
  Damper Const : Gain  Gain=c_Fuel
  Demux : Demux  Outputs=3
  Minus 1 to get Reaction Force : Gain  Gain=-1
  Product : Product
  Product1 : Product
  Spring Const : Gain  Gain=k_Fuel
  Sum : Sum  Inputs=+++
  Disturbance_y_b : Outport
  wires:
  Mass/1 -> Product/1
  Spring Const/1 -> Sum/1
  Damper Const/1 -> Sum/2
  Product/1 -> Sum/3
  Sum/1 -> Product1/1
  Arm_length r/1 -> Product1/2
  Product1/1 -> Minus 1 to get Reaction Force/1
  Minus 1 to get Reaction Force/1 -> Disturbance_y_b/1
  "Ang, d, 2d"/1 -> Demux/1
  Demux/1 -> Spring Const/1  "phi"
  Demux/2 -> Damper Const/1  "Phi_d"
  Demux/3 -> Product/2  "Phi_2d"

== matlab function MAIN/Plant/Forces)b/Engine/MATLAB Function ==
  data: phi input; Thrust_unit_vec output; theta input
function Thrust_unit_vec = fcn(phi, theta)
% Angles are defined to be the angle deflection ofthe thrust vector from 
% fixed z axis.  Right handed rotation used. 
% Sequence,
% phi about x, roll
% theta about y pitch to arrive at final orientation of thrust.
% rot mat of Thrust Vec Orientation from body fixed is calculated below. 
% Thrust vector orientation is initially aligned with body fixed. z_hat)T.V
% will always point down. opposite to the actual thrust vector.
C_phi = [1     0        0
         0 cos(phi) sin(phi) 
         0 -sin(phi) cos(phi)];

C_theta = [cos(theta) 0 -sin(theta)
           0          1           0
           sin(theta) 0 cos(theta)];

C_trans = C_theta * C_phi; % Thrust Fixed frame from body fixed

Thrust_unit_vec = C_trans.' * [0; 0; -1];% In Body Fixed
end

== matlab function MAIN/Visuals/Coord Transforms/Generalized Principle Axis and Angle of Rotation ==
  data: A output; RotMat input; phi output
function [A, phi] = fcn(RotMat)
% Rotation algorithms obtained form "Spacecraft Dynamics & Control (ARO
% 4090 text) pg 21 
phi = acos((trace(RotMat) -  1)/2); % eq 1.27
A = 1/(sin(phi)) * [RotMat(2,3) - RotMat(3,2)
                    RotMat(3,1) - RotMat(1,3)
                    RotMat(1,2) - RotMat(2,1)]; % eq 1.28

== matlab function MAIN/Visuals/Coord Transforms/NED Euler to VR Euler ==
  data: eu input; C output
function C = fcn(eu)
psi = eu(1); % FIrst rotation about NEDbody Fixed x
theta = eu(2); % Second rot about NEd Body fixed y
phi = eu(3); % Second rotation about NedBody Fixed Z

alpha =  -psi; % First rot about VR Body Fixed
beta = theta; % Second rotation about VR Body Fixed
gamm = -phi; % Thirst rot about VR Body fixed
 
Cz = [cos(alpha)  sin(alpha) 0
      -sin(alpha) cos(alpha) 0
      0           0          1];
Cx = [1 0         0
      0 cos(beta)  sin(beta)
      0 -sin(beta) cos(beta)];
Cy = [cos(gamm) 0 -sin(gamm)
      0         1 0
      sin(gamm) 0 cos(gamm)];
C = Cy * Cx * Cz;

== matlab function MAIN/Scope/rad2deg ==
  data: u input; y output
function y = fcn(u)

y = rad2deg(u);
